simulink model "SSModel_SIUnits"  (R2020b)
settings: Solver=VariableStepAuto  StartTime=0.0  StopTime=100  RelTol=1e-3
libraries: PB_Library_Master x1
settings Model: Creator=gfretti  LastModifiedBy=nbutler2
settings SFSimCC: CustomCodeUndefinedFunction=UseInterfaceOnly

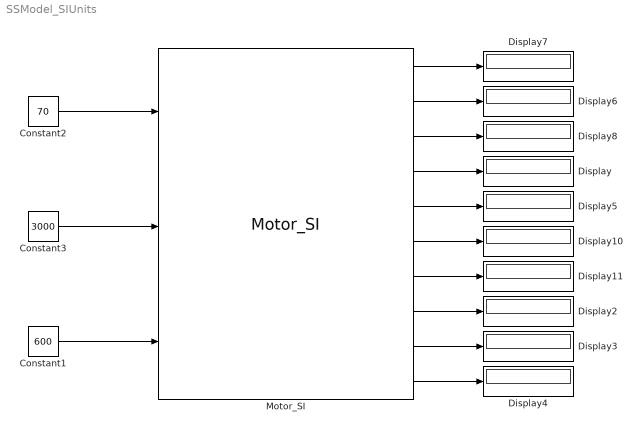
== system SSModel_SIUnits ==
  Constant1 : Constant  Value=600
  Constant2 : Constant  Value=70
  Constant3 : Constant  Value=3000
  Display{,2..8,10..11} (10 alike) : Display
  Motor_SI : PB_Library_Master/Motor_SI  pp=2.5  flux_m=0.46219  R_s=0.032  L_s=0.00115  P_Fe_Nom=904.3614  S_nom=3000  T_nom=70  P_out_max=22000  I_max=36.5  P_in_max=30000  T_max=80  MassEst_M=136.5892  Poles_i=5  R_s_i=.032  L_s_i=.00086+0.00029  S_nom_i=3000  T_nom_i=70  P_out_max_i=22000  I_max_i=36.5  P_in_max_i=30000  K_i=121  V_nom_i=368  T_max_i=80  CalculatePFe=Compute iron losses automatically  P_Fe_Nom_i=0  I_nom_i=36.5  PF_nom_i=0.99  P_Fe_Calc_Flag=1
  wires:
  Constant2/1 -> Motor_SI/1
  Constant1/1 -> Motor_SI/3
  Motor_SI/4 -> Display/1
  Motor_SI/8 -> Display2/1
  Motor_SI/9 -> Display3/1
  Motor_SI/10 -> Display4/1
  Motor_SI/5 -> Display5/1
  Motor_SI/2 -> Display6/1
  Motor_SI/1 -> Display7/1
  Motor_SI/3 -> Display8/1
  Motor_SI/6 -> Display10/1
  Constant3/1 -> Motor_SI/2
  Motor_SI/7 -> Display11/1
